simulink model "AttitudeComplementary2"  (Simulink 6.6)
settings: Solver=ode4  StartTime=0.0  StopTime=80  FixedStep=SampleT  RelTol=1e-3
InitFcn:
  | clc
  | Taxi_Var_new
  | failures
  | insInit
  | piccolo_init
values from neighbouring files (symbols this model uses):
  A1 = 0    [Taxi_Var.m]    (also in Taxi_Var_new.m = 0.007)
  Apolar = 0.0899    [Taxi_Var.m]    (also in Taxi_Var_new.m = 0.057)
  APtsamp = 0.005    [failures.m]    (also in piccolo_init.m = 0.05)
  CD0 = 0.0219    [Taxi_Var.m]    (also in Taxi_Var_new.m = 0.022)
  chord = S/span    (= 0.384036716878)    [Taxi_Var.m]    (also in Taxi_Var_new.m = 0.351341681574)
  CL0 = 0.1857    [Taxi_Var.m]    (also in Taxi_Var_new.m = 0.38)
  CLa = 4.6206    [Taxi_Var.m]    (also in Taxi_Var_new.m = 18.5)
  CLa_dot = 1.93    [Taxi_Var.m]    (also in Taxi_Var_new.m = 2.64)
  Clb = -0.0043    [Taxi_Var.m]    (also in Taxi_Var_new.m = -0.06)
  ClDa = 0.1695    [Taxi_Var.m]    (also in Taxi_Var_new.m)
  CLDe = 0.4032    [Taxi_Var.m]    (also in Taxi_Var_new.m = 0.24)
  CLDf = 0.047    [Taxi_Var.m]    (also in Taxi_Var_new.m = 0.4)
  ClDr = 0.0003    [Taxi_Var.m]    (also in Taxi_Var_new.m = 0.055)
  Clp = -0.4425    [Taxi_Var.m]    (also in Taxi_Var_new.m = -0.88)
  CLq = 8.7465    [Taxi_Var.m]    (also in Taxi_Var_new.m = 7.4)
  Clr = 0.0675    [Taxi_Var.m]    (also in Taxi_Var_new.m = 0.04)
  Cm0 = -0.0902    [Taxi_Var.m]    (also in Taxi_Var_new.m = 0.56)
  Cma = -1.3995    [Taxi_Var.m]    (also in Taxi_Var_new.m = -1.58)
  CmDe = -0.9493    [Taxi_Var.m]    (also in Taxi_Var_new.m = -41)
  CmDf = -.021    (= -0.021)    [Taxi_Var.m]    (also in Taxi_Var_new.m)
  Cmq = -10.8760    (= -10.876)    [Taxi_Var.m]    (also in Taxi_Var_new.m = -12)
  Cnb = 0.0281    [Taxi_Var.m]    (also in Taxi_Var_new.m = 0.73)
  CnDa = -0.0031    [Taxi_Var.m]    (also in Taxi_Var_new.m = -0.032)
  CnDr = -0.0882    [Taxi_Var.m]    (also in Taxi_Var_new.m = 0.19)
  Cnp = -0.0695    [Taxi_Var.m]    (also in Taxi_Var_new.m = -0.1)
  Cnr = -0.1045    [Taxi_Var.m]    (also in Taxi_Var_new.m = -0.23)
  CYb = -0.1999    [Taxi_Var.m]    (also in Taxi_Var_new.m = -0.98)
  CYDr = 0.0192    [Taxi_Var.m]    (also in Taxi_Var_new.m = 0.066)
  damax = 25*deg2rad    (= 0.436332312999)    [Taxi_Var.m]    (also in piccolo_init.m)
  damin = -25*deg2rad    (= -0.436332312999)    [Taxi_Var.m]    (also in piccolo_init.m)
  datrim = 0*deg2rad    (= 0)    [Taxi_Var.m]    (also in piccolo_init.m)
  demax = 15*deg2rad    (= 0.261799387799)    [Taxi_Var.m]    (also in piccolo_init.m)
  demin = -15*deg2rad    (= -0.261799387799)    [Taxi_Var.m]    (also in piccolo_init.m)
  detrim = -2.4137*deg2rad    (= -0.0421270121554)    [Taxi_Var.m]    (also in piccolo_init.m = -0.01308996939)
  dfland = 30*deg2rad    (= 0.523598775598)    [Taxi_Var.m]    (also in piccolo_init.m)
  dfmax = 30*deg2rad    (= 0.523598775598)    [Taxi_Var.m]    (also in piccolo_init.m)
  dfmin = 0*deg2rad    (= 0)    [Taxi_Var.m]    (also in piccolo_init.m)
  drmax = 25*deg2rad    (= 0.436332312999)    [Taxi_Var.m]    (also in piccolo_init.m)
  drmin = -25*deg2rad    (= -0.436332312999)    [Taxi_Var.m]    (also in piccolo_init.m)
  drtrim = 0*deg2rad    (= 0)    [Taxi_Var.m]    (also in piccolo_init.m)
  dtmax = 1    [Taxi_Var.m]    (also in piccolo_init.m)
  dtmin = 0    [Taxi_Var.m]    (also in piccolo_init.m)
  dttrim = 0.0725    [Taxi_Var.m]    (also in piccolo_init.m = 0.35)
  Euler_0 = [0; 0; 45]'*pi/180    [Taxi_Var.m]    (also in Taxi_Var_new.m = [0 0 45]'*pi/180)
  heightDown = 0    [insInit.m]
  heightUp = 3000    [insInit.m]
  IdxCmdOrbitRadius = 17    [piccolo_init.m]
  IdxCmdOrbitSense = 18    [piccolo_init.m]
  IdxCmdWp1Alt = 13    [piccolo_init.m]
  IdxCmdWp1Lat = 11    [piccolo_init.m]
  IdxCmdWp1Lon = 12    [piccolo_init.m]
  IdxCmdWp2Alt = 16    [piccolo_init.m]
  IdxCmdWp2Lat = 14    [piccolo_init.m]
  IdxCmdWp2Lon = 15    [piccolo_init.m]
  IdxEstimReserved1 = 4    [piccolo_init.m]
  IdxEstimWEast = 3    [piccolo_init.m]
  IdxEstimWNorth = 2    [piccolo_init.m]
  IdxGainsAltD = 10    [piccolo_init.m]
  IdxGainsAltI = 9    [piccolo_init.m]
  IdxGainsAltP = 8    [piccolo_init.m]
  IdxGainsPdynD = 4    [piccolo_init.m]
  IdxGainsPdynI = 3    [piccolo_init.m]
  IdxGainsPdynP = 2    [piccolo_init.m]
  IdxGainsPitchD = 7    [piccolo_init.m]
  IdxGainsPitchI = 6    [piccolo_init.m]
  IdxGainsPitchP = 5    [piccolo_init.m]
  IdxGainsRollD = 17    [piccolo_init.m]
  IdxGainsRollI = 16    [piccolo_init.m]
  IdxGainsRollP = 15    [piccolo_init.m]
  IdxGainsSlopeElevatorD = 25    [piccolo_init.m]
  IdxGainsSlopeElevatorP = 26    [piccolo_init.m]
  IdxGainsTrackConv = 24    [piccolo_init.m]
  IdxGainsTrackD = 23    [piccolo_init.m]
  IdxGainsTrackI = 22    [piccolo_init.m]
  IdxGainsTrackP = 21    [piccolo_init.m]
  IdxGainsTurnD = 14    [piccolo_init.m]
  IdxGainsTurnI = 13    [piccolo_init.m]
  IdxGainsTurnP = 12    [piccolo_init.m]
  IdxGainsYawD = 20    [piccolo_init.m]
  IdxGainsYawI = 19    [piccolo_init.m]
  IdxGainsYawP = 18    [piccolo_init.m]
  IdxLimitsAileronMax = 11    [piccolo_init.m]
  IdxLimitsAileronMin = 10    [piccolo_init.m]
  IdxLimitsBankMax = 9    [piccolo_init.m]
  IdxLimitsBankMin = 8    [piccolo_init.m]
  IdxLimitsElevatorMax = 13    [piccolo_init.m]
  IdxLimitsElevatorMin = 12    [piccolo_init.m]
  IdxLimitsFlapMax = 19    [piccolo_init.m]
  IdxLimitsFlapMin = 18    [piccolo_init.m]
  IdxLimitsPdynMax = 3    [piccolo_init.m]
  IdxLimitsPdynMin = 2    [piccolo_init.m]
  IdxLimitsRudderMax = 15    [piccolo_init.m]
  IdxLimitsRudderMin = 14    [piccolo_init.m]
  IdxLimitsThrottleMax = 17    [piccolo_init.m]
  IdxLimitsThrottleMin = 16    [piccolo_init.m]
  IdxSensorsAlt = 5    [piccolo_init.m]
  IdxSensorsLat = 3    [piccolo_init.m]
  IdxSensorsLon = 4    [piccolo_init.m]
  IdxSensorsVDown = 8    [piccolo_init.m]
  IdxSensorsVEast = 7    [piccolo_init.m]
  IdxSensorsVNorth = 6    [piccolo_init.m]
  IdxStatesGlobal = 2    [piccolo_init.m]
  IdxStatesManual = 16    [piccolo_init.m]
  IdxStatesMode = 15    [piccolo_init.m]
  ISA_g = 9.815    [Taxi_Var.m]    (also in Taxi_Var_new.m)
  ISA_hmax = 2000    [Taxi_Var.m]    (also in Taxi_Var_new.m)
  ISA_lapse = .0065    (= 0.0065)    [Taxi_Var.m]    (also in Taxi_Var_new.m)
  ISA_P0 = 101325    [Taxi_Var.m]    (also in Taxi_Var_new.m)
  ISA_R = 287    [Taxi_Var.m]    (also in Taxi_Var_new.m)
  ISA_rho0 = 1.225    [Taxi_Var.m]    (also in Taxi_Var_new.m)
  ISA_T0 = 289    [Taxi_Var.m]    (also in Taxi_Var_new.m)
  Ixx = 3.689084    [Taxi_Var.m]    (also in Taxi_Var_new.m = 3.8)
  Iyy = 7.43789    [Taxi_Var.m]    (also in Taxi_Var_new.m = 9.58)
  Izz = 10.22202    [Taxi_Var.m]    (also in Taxi_Var_new.m = 9.68)
  latDown = -100000    [insInit.m]
  latUp = 100000    [insInit.m]
  lonDown = -100000    [insInit.m]
  lonUp = 100000    [insInit.m]
  mass = 22.5    [Taxi_Var.m]    (also in Taxi_Var_new.m = 8.16466266)
  MinThK = 0.075    [Taxi_Var.m]    (also in Taxi_Var_new.m = 0.077)
  ... (+8 more)
undefined symbols (not defined in the file or in its folder): clock, DiscIntNeverNeededParam, Earth, gaind, polesd, WGS84, zerosd
libraries: piccolo_library x60, simulink x51, aerolibconvert2 x14, dspsigops x5, aerolibasang x5, aerolibatmos2 x2, aerolibtransform2 x2, aerolibnav x2, dspmtrx3 x1, aerolibutil x1
(part 4 of 6)

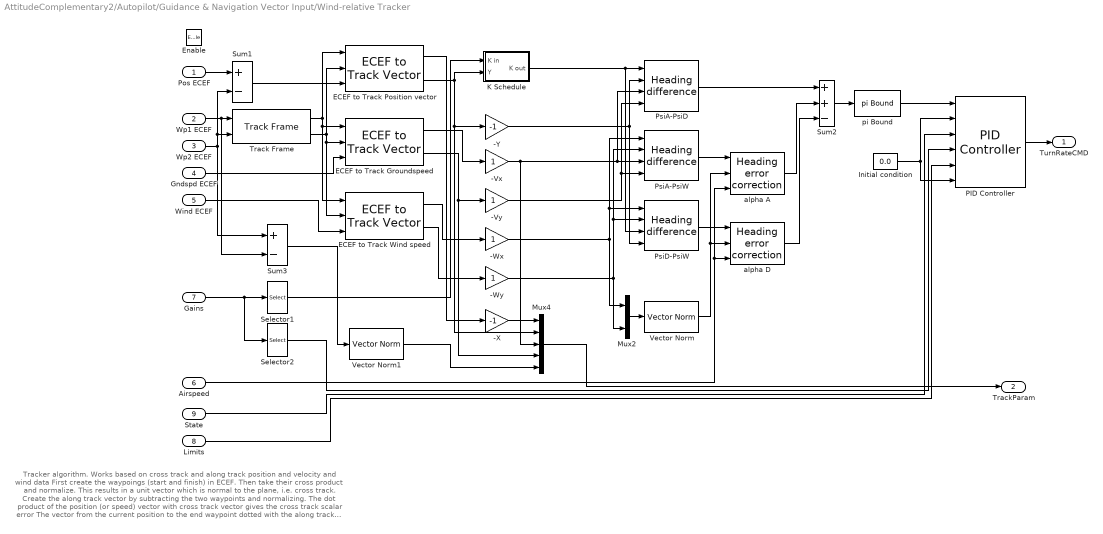
== system AttitudeComplementary2/Autopilot/Guidance & Navigation Vector Input/Wind-relative Tracker ==
  note: Tracker algorithm.  Works based on cross track and along track position and velocity and wind data
      |
      | First create the waypoings (start and finish) in ECEF.  Then take their cross product and normalize.  This results in a unit vector which is normal to the plane, i.e. cross track.
      | Create the along track vector by subtracting the two waypoints and normalizing.
      | The dot product of the position (or speed) vector with cross track vector gives the cross track scalar error
      | The vector from the current position to the end waypoint dotted with the along track vector gives the along track value
  Pos ECEF : Inport
  Wp1 ECEF : Inport  Port=2
  Wp2 ECEF : Inport  Port=3
  Gndspd ECEF : Inport  Port=4
  Wind ECEF : Inport  Port=5
  Airspeed : Inport  Port=6
  Gains : Inport  Port=7
  Limits : Inport  Port=8
  State : Inport  Port=9
  Enable : EnablePort
  -Vx : Gain  SaturateOnIntegerOverflow=on
  -Vy : Gain  SaturateOnIntegerOverflow=on
  -Wx : Gain  SaturateOnIntegerOverflow=on
  -Wy : Gain  SaturateOnIntegerOverflow=on
  -X : Gain  Gain=-1  SaturateOnIntegerOverflow=on
  -Y : Gain  Gain=-1  SaturateOnIntegerOverflow=on
  ECEF to Track Groundspeed : piccolo_library/Transformations/ECEF to Track Vector  SystemSampleTime=-1
  ECEF to Track Position vector : piccolo_library/Transformations/ECEF to Track Vector  SystemSampleTime=-1
  ECEF to Track Wind speed : piccolo_library/Transformations/ECEF to Track Vector  SystemSampleTime=-1
  Initial condition : Constant  Value=0.0
  K Schedule : Subsystem
  Mux2 : Mux  Inputs=2
  Mux4 : Mux  Inputs=5
  PID Controller : piccolo_library/Controllers/PID Controller  SystemSampleTime=-1  tsamp=tsamp  tdelay=tsamp
  PsiA-PsiD : piccolo_library/Controllers/Guidance/Heading difference  SystemSampleTime=-1
  PsiA-PsiW : piccolo_library/Controllers/Guidance/Heading difference  SystemSampleTime=-1
  PsiD-PsiW : piccolo_library/Controllers/Guidance/Heading difference  SystemSampleTime=-1
  Selector1 : Selector  IndexOptions=Index vector (dialog)  Indices=[4]  OutputSizes=1  InputPortWidth=4
  Selector2 : Selector  IndexOptions=Index vector (dialog)  Indices=[1 2 3]  OutputSizes=1  InputPortWidth=4
  Sum1 : Sum  Inputs=+-  SaturateOnIntegerOverflow=on  InputSameDT=on
  Sum2 : Sum  Inputs=++-  SaturateOnIntegerOverflow=on  InputSameDT=on
  Sum3 : Sum  Inputs=+-  SaturateOnIntegerOverflow=on  InputSameDT=on
  Track Frame : piccolo_library/Transformations/Track Frame  SystemSampleTime=-1
  Vector Norm : piccolo_library/Math/Vector Norm  SystemSampleTime=-1
  Vector Norm1 : piccolo_library/Math/Vector Norm  SystemSampleTime=-1
  alpha A : piccolo_library/Controllers/Guidance/Heading error correction  SystemSampleTime=-1
  alpha D : piccolo_library/Controllers/Guidance/Heading error correction  SystemSampleTime=-1
  pi Bound : piccolo_library/Math/pi Bound  SystemSampleTime=-1
  TurnRateCMD : Outport  OutDataType=fixdt(1,16,0)  OutScaling=[]
  TrackParam : Outport  Port=2  OutDataType=fixdt(1,16,0)  OutScaling=[]
  wires:
  Sum3/1 -> Vector Norm1/1
  Vector Norm1/1 -> Mux4/5
  -Y/1 -> PsiD-PsiW/4, PsiA-PsiD/2
  K Schedule/1(K out) -> PsiA-PsiD/1, PsiD-PsiW/3
  PID Controller/1 -> TurnRateCMD/1
  Initial condition/1 -> PID Controller/2, PID Controller/6
  -X/1 -> Mux4/1
  ECEF to Track Wind speed/1 -> -Wx/1
  ECEF to Track Wind speed/2 -> -Wy/1
  ECEF to Track Groundspeed/2 -> Mux4/4, -Vy/1
  ECEF to Track Groundspeed/1 -> -Vx/1
  ECEF to Track Position vector/1 -> -X/1
  ECEF to Track Position vector/2 -> -Y/1, Mux4/2, K Schedule/2(Y)
  Selector1/1 -> K Schedule/1(K in)
  Mux2/1 -> Vector Norm/1
  Vector Norm/1 -> alpha D/2, alpha A/2
  -Wy/1 -> Mux2/2, PsiD-PsiW/2, PsiA-PsiW/2
  -Vy/1 -> PsiA-PsiD/4, PsiA-PsiW/4
  -Wx/1 -> Mux2/1, PsiD-PsiW/1, PsiA-PsiW/1
  -Vx/1 -> Mux4/3, PsiA-PsiD/3, PsiA-PsiW/3
  pi Bound/1 -> PID Controller/1
  Sum2/1 -> pi Bound/1
  alpha D/1 -> Sum2/3
  alpha A/1 -> Sum2/2
  PsiA-PsiD/1 -> Sum2/1
  Limits/1 -> PID Controller/5
  State/1 -> PID Controller/3
  PsiD-PsiW/1 -> alpha D/1
  PsiA-PsiW/1 -> alpha A/1
  Mux4/1 -> TrackParam/1
  Selector2/1 -> PID Controller/4
  Airspeed/1 -> alpha D/3, alpha A/3
  Gains/1 -> Selector2/1, Selector1/1
  Wind ECEF/1 -> ECEF to Track Wind speed/3
  Gndspd ECEF/1 -> ECEF to Track Groundspeed/3
  Track Frame/2 -> ECEF to Track Wind speed/2, ECEF to Track Groundspeed/2, ECEF to Track Position vector/2
  Track Frame/1 -> ECEF to Track Wind speed/1, ECEF to Track Groundspeed/1, ECEF to Track Position vector/1
  Sum1/1 -> ECEF to Track Position vector/3
  Pos ECEF/1 -> Sum1/1
  Wp2 ECEF/1 -> Sum3/1, Sum1/2, Track Frame/2
  Wp1 ECEF/1 -> Sum3/2, Track Frame/1

== system AttitudeComplementary2/Autopilot/Pitch Control  Vector Inputs/PDynCmd ==
  AltError : Inport
  QCmd : Inport  Port=2
  QShift : Inport  Port=3
  QLimits : Inport  Port=4
  States : Inport  Port=5
  Density : Inport  Port=6
  -0.2 : Gain  Gain=-.2  SaturateOnIntegerOverflow=on
  0.3 : Gain  Gain=.3  SaturateOnIntegerOverflow=on
  1-based : Constant  Value=1.1
  All : Constant  Value=0
  Default : Constant  Value=0
  Enabled? : Logic  AllPortsSameDT=off
  Energy or not? : Switch  Threshold=0.5  SaturateOnIntegerOverflow=on
  Gravity : Gain  Gain=9.8  SaturateOnIntegerOverflow=on
  Lateral : Constant
  Limited QShift : piccolo_library/Nonlinear/SaturationEx  SystemSampleTime=-1
  Longitudinal : Constant  Value=0
  Manual assist switch : MultiPortSwitch  Inputs=5  SaturateOnIntegerOverflow=on  InputSameDT=on
  Mux : Mux  Inputs=2
  PDyn saturation : piccolo_library/Nonlinear/SaturationEx  SystemSampleTime=-1
  PDyn saturation1 : piccolo_library/Nonlinear/SaturationEx  SystemSampleTime=-1
  Qshift : Product  SaturateOnIntegerOverflow=on
  Selector1 : Selector  IndexOptions=Index vector (dialog)  Indices=IdxStatesManual  OutputSizes=1  InputPortWidth=SizeStates
  Selector2 : Selector  IndexOptions=Index vector (dialog)  Indices=IdxStatesAltToPdyn  OutputSizes=1  InputPortWidth=SizeStates
  Standard : Constant
  Sum : Sum  Inputs=|++  SaturateOnIntegerOverflow=on
  Sum1 : Sum  SaturateOnIntegerOverflow=on
  QCmdOut : Outport  OutDataType=fixdt(1,16,0)  OutScaling=[]
  QCmdNom : Outport  Port=2  OutDataType=fixdt(1,16,0)  OutScaling=[]
  wires:
  Enabled?/1 -> Energy or not?/2
  Manual assist switch/1 -> Enabled?/1
  Selector2/1 -> Enabled?/2
  PDyn saturation1/1 -> QCmdNom/1
  Sum1/1 -> PDyn saturation/1
  Energy or not?/1 -> Sum1/2
  QLimits/1 -> PDyn saturation1/2, PDyn saturation/2
  PDyn saturation/1 -> QCmdOut/1
  QShift/1 -> Energy or not?/3
  Limited QShift/1 -> Energy or not?/1
  Sum/1 -> Manual assist switch/1
  1-based/1 -> Sum/2
  Selector1/1 -> Sum/1
  States/1 -> Selector2/1, Selector1/1
  Default/1 -> Manual assist switch/6
  All/1 -> Manual assist switch/5
  Lateral/1 -> Manual assist switch/3
  Longitudinal/1 -> Manual assist switch/4
  Standard/1 -> Manual assist switch/2
  QCmd/1 -> PDyn saturation1/1, Sum1/1, -0.2/1, 0.3/1
  Qshift/1 -> Limited QShift/1
  Mux/1 -> Limited QShift/2
  0.3/1 -> Mux/2
  -0.2/1 -> Mux/1
  Gravity/1 -> Qshift/1
  AltError/1 -> Gravity/1
  Density/1 -> Qshift/2

== system AttitudeComplementary2/Autopilot/Pitch Control  Vector Inputs/Pdyn Hold ==
  Input : Inport
  Cmd : Inport  Port=2
  State : Inport  Port=3
  Gains : Inport  Port=4
  Limits : Inport  Port=5
  Actuator Trim : Inport  Port=6
  50 [Pa/s] : Constant  Value=100
  PID Controller : Subsystem  AncestorBlock=piccolo_library/Controllers/PID Controller  mask(PID Controller){tsamp=tsamp, tdelay=0.5}
      mask prompts: tsamp "Sample time:"; tdelay "Time derivative delay:"
      mask help: Generic PID (proportional, integral, derivative) controller with a single input and a single output.
  Rate Limit Ex : piccolo_library/Nonlinear/Rate Limit Ex  SystemSampleTime=-1  T=tsamp
  Out : Outport  OutDataType=fixdt(1,16,0)  OutScaling=[]
  wires:
  Actuator Trim/1 -> PID Controller/6(IniCond)
  Limits/1 -> PID Controller/5(Limits)
  Gains/1 -> PID Controller/4(Gains)
  State/1 -> PID Controller/3(State)
  PID Controller/1(Output) -> Out/1
  Rate Limit Ex/1 -> PID Controller/2(Cmd)
  Input/1 -> PID Controller/1(Input)
  50 [Pa/s]/1 -> Rate Limit Ex/2
  Cmd/1 -> Rate Limit Ex/1

== system AttitudeComplementary2/Autopilot/Pitch Control  Vector Inputs/Pitch Angle Hold ==
  note: Controller which takes in pitch rate and pitch angle and outputs elevator. The integral term is not used. Yet.
  Pitch angle : Inport
  Pitch rate : Inport  Port=2
  Pitch angle cmd : Inport  Port=3
  Pitch rate cmd : Inport  Port=4
  State : Inport  Port=5
  Gains : Inport  Port=6
  Demux1 : Demux  Outputs=3
  Demux5 : Demux  Outputs=3
  Derivative Gain : Product  Inputs=3  SaturateOnIntegerOverflow=on  InputSameDT=on
  Low-pass Filter : piccolo_library/Filters/Low-pass Filter  SystemSampleTime=-1  f=3  t=tsamp
  Proportional Gain : Product  Inputs=3  SaturateOnIntegerOverflow=on  InputSameDT=on
  Scope : Scope  NumInputPorts=5
      settings: YMin=-1~-0.075~-0.075~-5e+006~-5e+006  YMax=1~0.1~0.1~3.5e+007~3.5e+007  SaveName=ScopeData5
  Sum : Sum  SaturateOnIntegerOverflow=on  InputSameDT=on
  Sum1 : Sum  Inputs=|+-  SaturateOnIntegerOverflow=on  InputSameDT=on
  Sum2 : Sum  Inputs=|+-  SaturateOnIntegerOverflow=on  InputSameDT=on
  Terminator : Terminator
  Terminator1 : Terminator
  Out : Outport  OutDataType=fixdt(1,16,0)  OutScaling=[]
  wires:
  Demux1/2 -> Terminator1/1
  Demux1/1 -> Proportional Gain/3
  Demux1/3 -> Derivative Gain/3
  State/1 -> Demux1/1
  Demux5/2 -> Terminator/1
  Sum/1 -> Out/1, Scope/4
  Derivative Gain/1 -> Sum/2
  Proportional Gain/1 -> Sum/1, Scope/5
  Demux5/3 -> Derivative Gain/2
  Low-pass Filter/1 -> Derivative Gain/1
  Demux5/1 -> Proportional Gain/2
  Sum2/1 -> Proportional Gain/1, Scope/3
  Sum1/1 -> Low-pass Filter/1
  Pitch angle cmd/1 -> Sum2/2, Scope/1
  Pitch angle/1 -> Sum2/1, Scope/2
  Gains/1 -> Demux5/1
  Pitch rate/1 -> Sum1/1
  Pitch rate cmd/1 -> Sum1/2

== system AttitudeComplementary2/Autopilot/Roll Control Vector Inputs/Bank Angle Hold ==
  note: Controller which takes in roll rate and roll angle and outputs aileron.  Note that the derivative
      | term is simply the roll rate rather than the derivative of the error signal.
      | This is for backward compatible systems which aren't using the attitude data.
  note: pid
  Roll Rate : Inport
  Roll Angle : Inport  Port=2
  Cmd : Inport  Port=3
  State : Inport  Port=4
  Gains : Inport  Port=5
  Limits : Inport  Port=6
  IniCond : Inport  Port=7
  Demux1 : Demux  Outputs=3
  Demux2 : Demux  Outputs=3
  Derivative Gain : Product  Inputs=3  SaturateOnIntegerOverflow=on  InputSameDT=on
  Extended Integrator : piccolo_library/Integrators/Extended Integrator  SystemSampleTime=-1  T=tsamp
  Low-pass Filter : piccolo_library/Filters/Low-pass Filter  SystemSampleTime=-1  f=3  t=tsamp
  Proportional Gain : Product  Inputs=3  SaturateOnIntegerOverflow=on  InputSameDT=on
  Scope : Scope  NumInputPorts=10
      settings: YMin=-1~-0.07~-0.07~-0.02~-1~-1~-1~-1~-1~-1  YMax=1~0.03~0.03~0.07~1~1~1~1~1~1
  Sum2 : Sum  Inputs=+++  SaturateOnIntegerOverflow=on  InputSameDT=on
  Sum3 : Sum  Inputs=|+-  SaturateOnIntegerOverflow=on  InputSameDT=on
  Out : Outport  OutDataType=fixdt(1,16,0)  OutScaling=[]
  wires:
  Demux2/3 -> Derivative Gain/3
  Demux2/2 -> Extended Integrator/3
  Demux2/1 -> Proportional Gain/3
  State/1 -> Demux2/1
  Roll Rate/1 -> Low-pass Filter/1
  Low-pass Filter/1 -> Derivative Gain/1
  Demux1/2 -> Extended Integrator/4
  Sum2/1 -> Out/1, Scope/4
  Derivative Gain/1 -> Sum2/3, Scope/6  "derv"
  Extended Integrator/1 -> Sum2/2, Scope/5  "int"
  Proportional Gain/1 -> Sum2/1
  Demux1/3 -> Derivative Gain/2
  Demux1/1 -> Proportional Gain/2
  Limits/1 -> Extended Integrator/5
  IniCond/1 -> Extended Integrator/2
  Sum3/1 -> Extended Integrator/1, Proportional Gain/1, Scope/3  "err"
  Gains/1 -> Demux1/1
  Roll Angle/1 -> Scope/2, Sum3/1  "roll"
  Cmd/1 -> Sum3/2, Scope/1  "cmd"

== system AttitudeComplementary2/Autopilot/Roll Control Vector Inputs/Damper switch ==
  note: Select whether the individual components of the pitch and roll damper  loops are enabled or disabled.
      | This is done based on the specific loop enable state, the global state, and the mode of the autopilot.
      |
      | Note the use of the multiport  switch.  This switch is one based, and will truncate floating point
      | numbers.  Hence we add by 1.1 to guarantee we don't get the wrong state based on rounding
      | error.
  Globals : Inport
  Loop : Inport  Port=2
  Climbout : Constant
  Convert to 1 based : Constant  Value=1.1
  Default : Constant
  Demux : Demux  Outputs=3
  Display1 : Display
  Display2 : Display
  Display3 : Display
  Final Approach : Constant
  Flying : Constant
  Global and Loop on/off : Product  SaturateOnIntegerOverflow=on
  Land pattern : Constant
  Loop on or off : Switch  Threshold=0.5  SaturateOnIntegerOverflow=on
  Mux : Mux  Inputs=3
  Mux1 : Mux  Inputs=3
  Pre launch : Constant  Value=0
  Proportional\ Integral switch : MultiPortSwitch  Inputs=8  SaturateOnIntegerOverflow=on  InputSameDT=on
  Sum : Sum  Inputs=++|  SaturateOnIntegerOverflow=on  InputSameDT=on
  Terminator : Terminator
  Touchdown : Constant
  Transition : Constant  Value=0
  Zero : Constant  Value=0
  TriOut : Outport  OutDataType=fixdt(1,16,0)  OutScaling=[]
  wires:
  Default/1 -> Proportional\ Integral switch/9
  Touchdown/1 -> Proportional\ Integral switch/8
  Demux/3 -> Terminator/1
  Mux1/1 -> Loop on or off/1
  Proportional\ Integral switch/1 -> Mux1/3, Mux1/2, Mux1/1
  Final Approach/1 -> Proportional\ Integral switch/7
  Land pattern/1 -> Proportional\ Integral switch/6
  Flying/1 -> Proportional\ Integral switch/5
  Transition/1 -> Proportional\ Integral switch/3
  Climbout/1 -> Proportional\ Integral switch/4
  Pre launch/1 -> Proportional\ Integral switch/2
  Convert to 1 based/1 -> Sum/1
  Demux/2 -> Sum/2
  Sum/1 -> Proportional\ Integral switch/1
  Global and Loop on/off/1 -> Loop on or off/2, Display2/1
  Loop/1 -> Global and Loop on/off/2, Display3/1
  Demux/1 -> Global and Loop on/off/1, Display1/1
  Globals/1 -> Demux/1
  Zero/1 -> Mux/3, Mux/2, Mux/1
  Mux/1 -> Loop on or off/3
  Loop on or off/1 -> TriOut/1

== system AttitudeComplementary2/Autopilot/Roll Control Vector Inputs/Turn Rate Hold ==
  note: Standard PID feedback controller with integrator saturation. There are three gains, and three states, one for each term
  Input : Inport
  Cmd : Inport  Port=2
  State : Inport  Port=3
  Gains : Inport  Port=4
  Limits : Inport  Port=5
  IniCond : Inport  Port=6
  Demux : Demux  Outputs=3
  Demux1 : Demux  Outputs=3
  Derivative Gain : Product  Inputs=3  SaturateOnIntegerOverflow=on  InputSameDT=on
  Extended Integrator : piccolo_library/Integrators/Extended Integrator  SystemSampleTime=-1  T=tsamp
  Proportional Gain : Product  Inputs=3  SaturateOnIntegerOverflow=on  InputSameDT=on
  Scope1 : Scope  NumInputPorts=5
      settings: YMin=0.09325~0.09~-0.005~-1~-1  YMax=0.09475~0.1075~0.0125~1~1  SaveName=ScopeData25
  Sum : Sum  Inputs=|+-  SaturateOnIntegerOverflow=on
  Sum3 : Sum  Inputs=+++  SaturateOnIntegerOverflow=on  InputSameDT=on
  dx/dt with TD : piccolo_library/Derivatives/dx//dt with TD  SystemSampleTime=-1  tsamp=tsamp  tdelay=tdelay
  Output : Outport  OutDataType=fixdt(1,16,0)  OutScaling=[]
  wires:
  Sum3/1 -> Output/1, Scope1/4
  Demux1/3 -> Derivative Gain/3
  Demux1/2 -> Extended Integrator/3
  Demux1/1 -> Proportional Gain/3
  State/1 -> Demux1/1
  IniCond/1 -> Extended Integrator/2
  Limits/1 -> Extended Integrator/5
  Demux/2 -> Extended Integrator/4
  Extended Integrator/1 -> Sum3/2
  Derivative Gain/1 -> Sum3/3
  Proportional Gain/1 -> Sum3/1
  Demux/3 -> Derivative Gain/2
  Demux/1 -> Proportional Gain/2
  Gains/1 -> Demux/1
  dx/dt with TD/1 -> Derivative Gain/1
  Sum/1 -> Extended Integrator/1, dx/dt with TD/1, Scope1/3, Proportional Gain/1
  Cmd/1 -> Sum/2, Scope1/1
  Input/1 -> Sum/1, Scope1/2

== system AttitudeComplementary2/Get GPS in LTP/Geod2LTP2/ECEF2LTP (UEN) ==
  ECEF coordinates : Inport
  "Long, Lat" : Inport  Port=2
  Deg2R : Gain  Gain=pi/180  SaturateOnIntegerOverflow=on
  Demux3 : Demux  Outputs=2
  From Body to Universal1 : Subsystem
  Product1 : Product  Multiplication=Matrix(*)  SaturateOnIntegerOverflow=on  InputSameDT=on
  Out : Outport
  wires:
  "Long, Lat"/1 -> Deg2R/1
  Product1/1 -> Out/1
  Demux3/2 -> From Body to Universal1/2(lat)
  Demux3/1 -> From Body to Universal1/1(long)
  Deg2R/1 -> Demux3/1
  ECEF coordinates/1 -> Product1/2
  From Body to Universal1/1(DCM) -> Product1/1

== system AttitudeComplementary2/Get GPS in LTP/Geod2LTP2/Geod2ECEF ==
  "height, m" : Inport
  "lat, deg" : Inport  Port=2
  lon,deg : Inport  Port=3
  (Rh+h)cos(phi)*cos(lamb)=Xe : Product  Inputs=3  SaturateOnIntegerOverflow=on  InputSameDT=on
  (Rh+h)cos(phi)*sin(lamb)=Ye : Product  Inputs=3  SaturateOnIntegerOverflow=on  InputSameDT=on
  Deg2R : Gain  Gain=pi/180  SaturateOnIntegerOverflow=on
  "Deg2R " : Gain  Gain=pi/180  SaturateOnIntegerOverflow=on
  Product1 : Product  SaturateOnIntegerOverflow=on  InputSameDT=on
  Re=equatorial radius : Constant  Value=Re
  Rh : Product  Inputs=*/  SaturateOnIntegerOverflow=on  InputSameDT=on
  Rh(1-e^2) : Product  SaturateOnIntegerOverflow=on  InputSameDT=on
  Sum1 : Sum  Inputs=+-|  SaturateOnIntegerOverflow=on  InputSameDT=on
  Sum2 : Sum  SaturateOnIntegerOverflow=on  InputSameDT=on
      settings: AttributesFormatString=Rh+h
  Sum3 : Sum  Inputs=|+-  SaturateOnIntegerOverflow=on  InputSameDT=on
  Sum4 : Sum  SaturateOnIntegerOverflow=on  InputSameDT=on
      settings: AttributesFormatString=(1-e^2)Rh+h
  Ze : Product  SaturateOnIntegerOverflow=on  InputSameDT=on
  const : Constant
  const1 : Constant
  cos(lamb) : Trigonometry  Operator=cos
  cos(phi) : Trigonometry  Operator=cos
  eccentricity^2 : Subsystem
  f : Fcn  Expr=sqrt(u(1))
  sin(lamb) : Trigonometry
  sin(phi) : Trigonometry
  sin(phi)^2 : Product  SaturateOnIntegerOverflow=on  InputSameDT=on
  "Xe, m " : Outport
  "Ye, m " : Outport  Port=2
  "Ze, m " : Outport  Port=3
  wires:
  "lat, deg"/1 -> Deg2R/1
  sin(phi)/1 -> sin(phi)^2/1, sin(phi)^2/2, Ze/1
  f/1 -> Rh/2
  Re=equatorial radius/1 -> Rh/1
  Rh/1 -> Sum2/2, Rh(1-e^2)/2
  Product1/1 -> Sum1/2
  Sum1/1 -> f/1
  const/1 -> Sum1/1
  "height, m"/1 -> Sum4/2, Sum2/1
  eccentricity^2/1(e^2) -> Product1/1, Sum3/2
  sin(phi)^2/1 -> Product1/2
  const1/1 -> Sum3/1
  Sum3/1 -> Rh(1-e^2)/1  "1-e^2"
  Rh(1-e^2)/1 -> Sum4/1
  Sum4/1 -> Ze/2
  lon,deg/1 -> "Deg2R "/1
  cos(phi)/1 -> (Rh+h)cos(phi)*cos(lamb)=Xe/2, (Rh+h)cos(phi)*sin(lamb)=Ye/2
  cos(lamb)/1 -> (Rh+h)cos(phi)*cos(lamb)=Xe/3
  sin(lamb)/1 -> (Rh+h)cos(phi)*sin(lamb)=Ye/3
  Ze/1 -> "Ze, m "/1
  Deg2R/1 -> cos(phi)/1, sin(phi)/1
  "Deg2R "/1 -> cos(lamb)/1, sin(lamb)/1
  Sum2/1 -> (Rh+h)cos(phi)*sin(lamb)=Ye/1, (Rh+h)cos(phi)*cos(lamb)=Xe/1
  (Rh+h)cos(phi)*cos(lamb)=Xe/1 -> "Xe, m "/1
  (Rh+h)cos(phi)*sin(lamb)=Ye/1 -> "Ye, m "/1

== system AttitudeComplementary2/Get GPS in LTP/Geod2LTP2/Geod2ECEF1 ==
  "height, m" : Inport
  "lat, deg" : Inport  Port=2
  lon,deg : Inport  Port=3
  (Rh+h)cos(phi)*cos(lamb)=Xe : Product  Inputs=3  SaturateOnIntegerOverflow=on  InputSameDT=on
  (Rh+h)cos(phi)*sin(lamb)=Ye : Product  Inputs=3  SaturateOnIntegerOverflow=on  InputSameDT=on
  Deg2R : Gain  Gain=pi/180  SaturateOnIntegerOverflow=on
  "Deg2R " : Gain  Gain=pi/180  SaturateOnIntegerOverflow=on
  Product1 : Product  SaturateOnIntegerOverflow=on  InputSameDT=on
  Re=equatorial radius : Constant  Value=Re
  Rh : Product  Inputs=*/  SaturateOnIntegerOverflow=on  InputSameDT=on
  Rh(1-e^2) : Product  SaturateOnIntegerOverflow=on  InputSameDT=on
  Sum1 : Sum  Inputs=+-|  SaturateOnIntegerOverflow=on  InputSameDT=on
  Sum2 : Sum  SaturateOnIntegerOverflow=on  InputSameDT=on
      settings: AttributesFormatString=Rh+h
  Sum3 : Sum  Inputs=|+-  SaturateOnIntegerOverflow=on  InputSameDT=on
  Sum4 : Sum  SaturateOnIntegerOverflow=on  InputSameDT=on
      settings: AttributesFormatString=(1-e^2)Rh+h
  Ze : Product  SaturateOnIntegerOverflow=on  InputSameDT=on
  const : Constant
  const1 : Constant
  cos(lamb) : Trigonometry  Operator=cos
  cos(phi) : Trigonometry  Operator=cos
  eccentricity^2 : Subsystem
  f : Fcn  Expr=sqrt(u(1))
  sin(lamb) : Trigonometry
  sin(phi) : Trigonometry
  sin(phi)^2 : Product  SaturateOnIntegerOverflow=on  InputSameDT=on
  "Xe, m " : Outport
  "Ye, m " : Outport  Port=2
  "Ze, m " : Outport  Port=3
  wires:
  (Rh+h)cos(phi)*sin(lamb)=Ye/1 -> "Ye, m "/1
  (Rh+h)cos(phi)*cos(lamb)=Xe/1 -> "Xe, m "/1
  Sum2/1 -> (Rh+h)cos(phi)*cos(lamb)=Xe/1, (Rh+h)cos(phi)*sin(lamb)=Ye/1
  "Deg2R "/1 -> sin(lamb)/1, cos(lamb)/1
  Deg2R/1 -> sin(phi)/1, cos(phi)/1
  Ze/1 -> "Ze, m "/1
  sin(lamb)/1 -> (Rh+h)cos(phi)*sin(lamb)=Ye/3
  cos(lamb)/1 -> (Rh+h)cos(phi)*cos(lamb)=Xe/3
  cos(phi)/1 -> (Rh+h)cos(phi)*sin(lamb)=Ye/2, (Rh+h)cos(phi)*cos(lamb)=Xe/2
  lon,deg/1 -> "Deg2R "/1
  Sum4/1 -> Ze/2
  Rh(1-e^2)/1 -> Sum4/1
  Sum3/1 -> Rh(1-e^2)/1  "1-e^2"
  const1/1 -> Sum3/1
  sin(phi)^2/1 -> Product1/2
  eccentricity^2/1(e^2) -> Sum3/2, Product1/1
  "height, m"/1 -> Sum2/1, Sum4/2
  const/1 -> Sum1/1
  Sum1/1 -> f/1
  Product1/1 -> Sum1/2
  Rh/1 -> Rh(1-e^2)/2, Sum2/2
  Re=equatorial radius/1 -> Rh/1
  f/1 -> Rh/2
  sin(phi)/1 -> Ze/1, sin(phi)^2/2, sin(phi)^2/1
  "lat, deg"/1 -> Deg2R/1

== system AttitudeComplementary2/Gyro Comp/3vector LPF/Low Pass1 ==
  In1 : Inport
  Discrete Zero-Pole : DiscreteZeroPole  Zeros=zerosd  Poles=polesd  Gain=gaind  SampleTime=SampleTime
  Out1 : Outport
  wires:
  In1/1 -> Discrete Zero-Pole/1
  Discrete Zero-Pole/1 -> Out1/1

== system AttitudeComplementary2/Gyro Comp/3vector LPF/Low Pass2 ==
  In1 : Inport
  Discrete Zero-Pole : DiscreteZeroPole  Zeros=zerosd  Poles=polesd  Gain=gaind  SampleTime=SampleTime
  Out1 : Outport
  wires:
  Discrete Zero-Pole/1 -> Out1/1
  In1/1 -> Discrete Zero-Pole/1

== system AttitudeComplementary2/Gyro Comp/3vector LPF/Low Pass3 ==
  In1 : Inport
  Discrete Zero-Pole : DiscreteZeroPole  Zeros=zerosd  Poles=polesd  Gain=gaind  SampleTime=SampleTime
  Out1 : Outport
  wires:
  In1/1 -> Discrete Zero-Pole/1
  Discrete Zero-Pole/1 -> Out1/1

== system AttitudeComplementary2/Interpolate Data/Subsystem/Clock Updates ==
  change? : Inport
  Constant : Constant
  Constant1 : Constant  Value=0
  Constant2 : Constant  Value=SampleT
  Discrete-Time Integrator : DiscreteIntegrator  ExternalReset=rising  InitialConditionSource=external  SampleTime=SampleT  ICPrevOutput=DiscIntNeverNeededParam  ICPrevScaledInput=DiscIntNeverNeededParam
  Integer Delay2 : simulink/Discrete/Integer Delay  vinit=0.0  samptime=-1  NumDelays=1
  Sum : Sum  Inputs=|++
  clock : Outport
  wires:
  Constant/1 -> Discrete-Time Integrator/1
  Constant1/1 -> Discrete-Time Integrator/3
  Discrete-Time Integrator/1 -> Integer Delay2/1
  change?/1 -> Discrete-Time Integrator/2
  Integer Delay2/1 -> Sum/1
  Constant2/1 -> Sum/2
  Sum/1 -> clock/1

== system AttitudeComplementary2/Interpolate Data/Subsystem/Detect Change ==
  Data : Inport
  Abs1 : Abs
  Difference1 : simulink/Discrete/Difference  SystemSampleTime=-1  ICPrevInput=0.0  OutDataType=sfix(16)  OutScaling=2^-10  DoSatur=off
  Saturation1 : Saturate  UpperLimit=1  LowerLimit=0  SampleTime=SampleT
  change? : Outport
  wires:
  Difference1/1 -> Abs1/1
  Abs1/1 -> Saturation1/1
  Data/1 -> Difference1/1
  Saturation1/1 -> change?/1

== system AttitudeComplementary2/Interpolate Data/Subsystem/Generate Clock ==
  Reset : Inport
  Constant : Constant
  Discrete-Time Integrator : DiscreteIntegrator  ExternalReset=rising  InitialConditionMode=State only (most efficient)  SampleTime=SampleT  ICPrevOutput=DiscIntNeverNeededParam  ICPrevScaledInput=DiscIntNeverNeededParam
  Rate Transition2 : RateTransition  OutPortSampleTime=SampleT
  Clock : Outport
  wires:
  Constant/1 -> Discrete-Time Integrator/1
  Rate Transition2/1 -> Discrete-Time Integrator/2
  Reset/1 -> Rate Transition2/1
  Discrete-Time Integrator/1 -> Clock/1

== system AttitudeComplementary2/Interpolate Data/Subsystem/Low Pass ==
  In1 : Inport
  Discrete Zero-Pole : DiscreteZeroPole  Zeros=zerosd  Poles=polesd  Gain=gaind  SampleTime=SampleTime
  Out1 : Outport
  wires:
  Discrete Zero-Pole/1 -> Out1/1
  In1/1 -> Discrete Zero-Pole/1

== system AttitudeComplementary2/Interpolate Data/Subsystem/Low Pass1 ==
  In1 : Inport
  Discrete Zero-Pole : DiscreteZeroPole  Zeros=zerosd  Poles=polesd  Gain=gaind  SampleTime=SampleTime
  Out1 : Outport
  wires:
  In1/1 -> Discrete Zero-Pole/1
  Discrete Zero-Pole/1 -> Out1/1

== system AttitudeComplementary2/Interpolate Data/Subsystem/Low Pass2 ==
  In1 : Inport
  Discrete Zero-Pole : DiscreteZeroPole  Zeros=zerosd  Poles=polesd  Gain=gaind  SampleTime=SampleTime
  Out1 : Outport
  wires:
  Discrete Zero-Pole/1 -> Out1/1
  In1/1 -> Discrete Zero-Pole/1

== system AttitudeComplementary2/Interpolate Data/Subsystem/SampleData ==
  data : Inport
  clock : Inport  Port=2
  Enable : EnablePort
  Integer Delay{,1..3} (4 alike) : simulink/Discrete/Integer Delay  vinit=0.0  samptime=-1  NumDelays=1
  k : Outport
  km1 : Outport  Port=2
  km2 : Outport  Port=3
  tm1 : Outport  Port=4
  tm2 : Outport  Port=5
  wires:
  data/1 -> Integer Delay/1, k/1
  Integer Delay/1 -> Integer Delay1/1, km1/1
  Integer Delay1/1 -> km2/1
  clock/1 -> Integer Delay2/1
  Integer Delay2/1 -> tm1/1, Integer Delay3/1
  Integer Delay3/1 -> tm2/1

== system AttitudeComplementary2/Interpolate Data/Subsystem1/Detect Change ==
  Data : Inport
  Abs1 : Abs
  Difference1 : simulink/Discrete/Difference  SystemSampleTime=-1  ICPrevInput=0.0  OutDataType=sfix(16)  OutScaling=2^-10  DoSatur=off
  Saturation1 : Saturate  UpperLimit=1  LowerLimit=0  SampleTime=SampleT
  change? : Outport
  wires:
  Saturation1/1 -> change?/1
  Data/1 -> Difference1/1
  Abs1/1 -> Saturation1/1
  Difference1/1 -> Abs1/1

== system AttitudeComplementary2/Interpolate Data/Subsystem1/Generate Clock ==
  Reset : Inport
  Constant : Constant
  Discrete-Time Integrator : DiscreteIntegrator  ExternalReset=rising  InitialConditionMode=State only (most efficient)  SampleTime=SampleT  ICPrevOutput=DiscIntNeverNeededParam  ICPrevScaledInput=DiscIntNeverNeededParam
  Rate Transition2 : RateTransition  OutPortSampleTime=SampleT
  Clock : Outport
  wires:
  Discrete-Time Integrator/1 -> Clock/1
  Reset/1 -> Rate Transition2/1
  Rate Transition2/1 -> Discrete-Time Integrator/2
  Constant/1 -> Discrete-Time Integrator/1

== system AttitudeComplementary2/Interpolate Data/Subsystem1/Low Pass ==
  In1 : Inport
  Discrete Zero-Pole : DiscreteZeroPole  Zeros=zerosd  Poles=polesd  Gain=gaind  SampleTime=SampleTime
  Out1 : Outport
  wires:
  In1/1 -> Discrete Zero-Pole/1
  Discrete Zero-Pole/1 -> Out1/1

== system AttitudeComplementary2/Interpolate Data/Subsystem1/Low Pass1 ==
  In1 : Inport
  Discrete Zero-Pole : DiscreteZeroPole  Zeros=zerosd  Poles=polesd  Gain=gaind  SampleTime=SampleTime
  Out1 : Outport
  wires:
  Discrete Zero-Pole/1 -> Out1/1
  In1/1 -> Discrete Zero-Pole/1

== system AttitudeComplementary2/Interpolate Data/Subsystem1/SampleData ==
  data : Inport
  Enable : EnablePort
  Integer Delay : simulink/Discrete/Integer Delay  vinit=0.0  samptime=-1  NumDelays=1
  Integer Delay1 : simulink/Discrete/Integer Delay  vinit=0.0  samptime=-1  NumDelays=1
  k : Outport
  km1 : Outport  Port=2
  km2 : Outport  Port=3
  wires:
  Integer Delay1/1 -> km2/1
  Integer Delay/1 -> km1/1, Integer Delay1/1
  data/1 -> k/1, Integer Delay/1

== system AttitudeComplementary2/Interpolate Data/Subsystem2/Detect Change ==
  Data : Inport
  Abs1 : Abs
  Difference1 : simulink/Discrete/Difference  SystemSampleTime=-1  ICPrevInput=0.0  OutDataType=sfix(16)  OutScaling=2^-10  DoSatur=off
  Saturation1 : Saturate  UpperLimit=1  LowerLimit=0  SampleTime=SampleT
  change? : Outport
  wires:
  Difference1/1 -> Abs1/1
  Abs1/1 -> Saturation1/1
  Data/1 -> Difference1/1
  Saturation1/1 -> change?/1

== system AttitudeComplementary2/Interpolate Data/Subsystem2/Generate Clock ==
  Reset : Inport
  Constant : Constant
  Discrete-Time Integrator : DiscreteIntegrator  ExternalReset=rising  InitialConditionMode=State only (most efficient)  SampleTime=SampleT  ICPrevOutput=DiscIntNeverNeededParam  ICPrevScaledInput=DiscIntNeverNeededParam
  Rate Transition2 : RateTransition  OutPortSampleTime=SampleT
  Clock : Outport
  wires:
  Constant/1 -> Discrete-Time Integrator/1
  Rate Transition2/1 -> Discrete-Time Integrator/2
  Reset/1 -> Rate Transition2/1
  Discrete-Time Integrator/1 -> Clock/1

== system AttitudeComplementary2/Interpolate Data/Subsystem2/Low Pass ==
  In1 : Inport
  Discrete Zero-Pole : DiscreteZeroPole  Zeros=zerosd  Poles=polesd  Gain=gaind  SampleTime=SampleTime
  Out1 : Outport
  wires:
  Discrete Zero-Pole/1 -> Out1/1
  In1/1 -> Discrete Zero-Pole/1

== system AttitudeComplementary2/Interpolate Data/Subsystem2/Low Pass1 ==
  In1 : Inport
  Discrete Zero-Pole : DiscreteZeroPole  Zeros=zerosd  Poles=polesd  Gain=gaind  SampleTime=SampleTime
  Out1 : Outport
  wires:
  In1/1 -> Discrete Zero-Pole/1
  Discrete Zero-Pole/1 -> Out1/1

== system AttitudeComplementary2/Interpolate Data/Subsystem2/SampleData ==
  data : Inport
  Enable : EnablePort
  Integer Delay : simulink/Discrete/Integer Delay  vinit=0.0  samptime=-1  NumDelays=1
  Integer Delay1 : simulink/Discrete/Integer Delay  vinit=0.0  samptime=-1  NumDelays=1
  k : Outport
  km1 : Outport  Port=2
  km2 : Outport  Port=3
  wires:
  data/1 -> Integer Delay/1, k/1
  Integer Delay/1 -> Integer Delay1/1, km1/1
  Integer Delay1/1 -> km2/1

== system AttitudeComplementary2/L1 Adaptive Controller LATERAL-DIRECTIONAL/PF Yaw Channel L1 Augmentation/Adaptive Law ==
  u_psi_tilda : Inport
  Integrator : Integrator  LimitOutput=on  UpperSaturationLimit=Pbound  LowerSaturationLimit=-Pbound
  ON : Constant  Value=gamma
  Projection : Product  RndMeth=Zero
  Scope1 : Scope  NumInputPorts=3
      settings: YMin=-0.1~-0.004~-6  YMax=0.1~0.003~8  SaveName=ScopeData27
  sighat_2 : Outport
  wires:
  Integrator/1 -> sighat_2/1, Scope1/1
  ON/1 -> Projection/1
  Projection/1 -> Integrator/1, Scope1/3
  u_psi_tilda/1 -> Projection/2, Scope1/2  "u_psi_tilda"

== system AttitudeComplementary2/L1 Adaptive Controller LATERAL-DIRECTIONAL/PF Yaw Channel L1 Augmentation/C(s) ==
  sighat_2 : Inport
  Integrator2 : Integrator
  ON : Constant  Value=omega
  Product : Product  RndMeth=Zero
  Sum2 : Sum  Inputs=|+-
  C_sighat_2 : Outport
  wires:
  Integrator2/1 -> C_sighat_2/1, Sum2/2
  Sum2/1 -> Product/2
  Product/1 -> Integrator2/1
  sighat_2/1 -> Sum2/1
  ON/1 -> Product/1

== system AttitudeComplementary2/L1 Adaptive Controller LATERAL-DIRECTIONAL/PF Yaw Channel L1 Augmentation/State predictor ==
  u2 : Inport
  sighat_2 : Inport  Port=2
  Integrator2 : Integrator
  ON : Constant  Value=m
  Product : Product  RndMeth=Zero
  Sum1 : Sum  Inputs=|++
  Sum2 : Sum  Inputs=|+-
  u_psi_hat : Outport
  wires:
  sighat_2/1 -> Sum1/2
  Sum1/1 -> Sum2/1
  u2/1 -> Sum1/1
  Integrator2/1 -> u_psi_hat/1, Sum2/2
  Sum2/1 -> Product/2
  Product/1 -> Integrator2/1
  ON/1 -> Product/1

== system AttitudeComplementary2/L1 Adaptive Controller LONGITUDINAL/PF Yaw Channel L1 Augmentation/Adaptive Law ==
  u_psi_tilda : Inport
  Integrator : Integrator  LimitOutput=on  UpperSaturationLimit=Pbound  LowerSaturationLimit=-Pbound
  ON : Constant  Value=gamma
  Projection : Product  RndMeth=Zero
  Scope1 : Scope  NumInputPorts=3
      settings: TimeRange=4  YMin=-0.1~-1000~-6  YMax=0.1~200~8  SaveName=ScopeData27
  sighat_2 : Outport
  wires:
  u_psi_tilda/1 -> Scope1/2, Projection/2  "u_psi_tilda"
  Projection/1 -> Scope1/3, Integrator/1
  ON/1 -> Projection/1
  Integrator/1 -> Scope1/1, sighat_2/1

== system AttitudeComplementary2/L1 Adaptive Controller LONGITUDINAL/PF Yaw Channel L1 Augmentation/C(s) ==
  sighat_2 : Inport
  Integrator2 : Integrator
  ON : Constant  Value=omega
  Product : Product  RndMeth=Zero
  Sum2 : Sum  Inputs=|+-
  C_sighat_2 : Outport
  wires:
  ON/1 -> Product/1
  sighat_2/1 -> Sum2/1
  Product/1 -> Integrator2/1
  Sum2/1 -> Product/2
  Integrator2/1 -> Sum2/2, C_sighat_2/1

== system AttitudeComplementary2/L1 Adaptive Controller LONGITUDINAL/PF Yaw Channel L1 Augmentation/State predictor ==
  u2 : Inport
  sighat_2 : Inport  Port=2
  Integrator2 : Integrator
  ON : Constant  Value=m
  Product : Product  RndMeth=Zero
  Sum1 : Sum  Inputs=|++
  Sum2 : Sum  Inputs=|+-
  u_psi_hat : Outport
  wires:
  ON/1 -> Product/1
  Product/1 -> Integrator2/1
  Sum2/1 -> Product/2
  Integrator2/1 -> Sum2/2, u_psi_hat/1
  u2/1 -> Sum1/1
  Sum1/1 -> Sum2/1
  sighat_2/1 -> Sum1/2

== system AttitudeComplementary2/Plant Model/Plant/6-DOF EOM ==
  "[F,M]" : Inport
  Vb Corr : Inport  Orientation=left  Port=2
  Angular Rates : Integrator  InitialCondition=PQR_0'
  Demux1 : Demux  Outputs=[3 3]
  Euler Angles : Integrator  InitialCondition=Euler_0'
  Get Euler Dot : Subsystem
      mask Display:
      | port_label('input', 1, 'p, q, r')
      | port_label('input', 2, 'Euler')
      | port_label('output', 1, 'Euler_dot')
  Mux : Mux  Orientation=left  Inputs=[3;3]
  NED2NEU : Gain  Gain=[1 0 0;0 1 0;0 0 -1]  Multiplication=Matrix(K*u)  SaturateOnIntegerOverflow=on
  Position : Integrator  InitialCondition=Pos_0'
  RB2L * Vb : Product  Multiplication=Matrix(*)  SaturateOnIntegerOverflow=on  InputSameDT=on
  RB2LTP : Subsystem
  Velocities Body : Integrator  InitialCondition=Vb_0'
  "[V1,2,3,W1,2,3]" : Subsystem
  X,Y,Z (LTP) : Outport
  "Vx, Vy, Vz" : Outport  Port=2
  Euler : Outport  Port=3
  "p, q, r" : Outport  Orientation=left  Port=4
  Euler_dot : Outport  Port=5
  Vb : Outport  Port=6
  Ab : Outport  Port=7
  Ab meas : Outport  Port=8
  wires:
  "[V1,2,3,W1,2,3]"/1("Acc_meas ") -> Ab meas/1
  Euler Angles/1 -> "[V1,2,3,W1,2,3]"/2(Euler), Get Euler Dot/2(Euler), Euler/1, RB2LTP/1(Euler)
  Demux1/1 -> Ab/1, Velocities Body/1
  "[V1,2,3,W1,2,3]"/2(V*dot) -> Demux1/1
  Demux1/2 -> Angular Rates/1
  "[F,M]"/1 -> "[V1,2,3,W1,2,3]"/1("[F ; M]")
  RB2LTP/1(Rot) -> RB2L * Vb/1
  Velocities Body/1 -> Vb/1, RB2L * Vb/2
  Mux/1 -> "[V1,2,3,W1,2,3]"/3(V*)
  Position/1 -> X,Y,Z (LTP)/1
  Angular Rates/1 -> Get Euler Dot/1(p,q,r), Mux/2, "p, q, r"/1
  RB2L * Vb/1 -> NED2NEU/1, "Vx, Vy, Vz"/1  "NED"
  NED2NEU/1 -> Position/1
  Get Euler Dot/1(Euler_dot) -> Euler Angles/1, Euler_dot/1
  Vb Corr/1 -> Mux/1

== system AttitudeComplementary2/Plant Model/Plant/Engine Model ==
  dt : Inport
  Vmag : Inport  Port=2
  Constant4 : Constant  Value=0
  Get To1 : Subsystem
  Mux : Mux  Inputs=2
  Mux1 : Mux  Inputs=3
  Thrust Available (lbs) : Fcn  Expr=u(1) - 0.047*sqrt(u(1))*u(2)
  kg2N : Gain  Gain=ISA_g  SaturateOnIntegerOverflow=on
  lbs2kg : Gain  Gain=0.45359237  SaturateOnIntegerOverflow=on
  RPM : Outport
  Thrust : Outport  Port=2
  wires:
  Get To1/1(RPM) -> RPM/1
  dt/1 -> Get To1/1(dt)
  Get To1/2(To) -> Mux/1
  Mux/1 -> Thrust Available (lbs)/1
  Thrust Available (lbs)/1 -> lbs2kg/1
  Vmag/1 -> Mux/2
  Mux1/1 -> Thrust/1
  lbs2kg/1 -> kg2N/1
  Constant4/1 -> Mux1/2, Mux1/3
  kg2N/1 -> Mux1/1

== system AttitudeComplementary2/Plant Model/Plant/Forces and Moments ==
  Wind e : Inport
  Rho : Inport  Port=2
  "de, deg" : Inport  Port=3
  da,deg : Inport  Port=4
  "dr, deg" : Inport  Port=5
  "df, deg" : Inport  Port=6
  "Vx, Vy, Vz " : Inport  Port=7
  Euler : Inport  Port=8  PortDimensions=3
  p,q,r : Inport  Port=9
  Alpha/Beta : Subsystem
  Body Frame F & M : Subsystem
  Get Grav Force in Body : Subsystem
  Gravitational Force : Constant  Value=[0 0 mass*ISA_g]  VectorParams1D=off
  Mux : Mux  Inputs=2
  Mux1 : Mux  Inputs=2
  NED(u)2b : Subsystem
  Scope : Scope
      settings: SaveName=ScopeData5
  Selector : Selector  IndexOptions=Index vector (dialog)  Indices=3  OutputSizes=1  InputPortWidth=3
  Selector1 : Selector  Orientation=up  IndexOptions=Index vector (dialog)  Indices=3  OutputSizes=1  InputPortWidth=3
  Sum : Sum  Inputs=|++  SaturateOnIntegerOverflow=on
  Vair : Sum  Inputs=+-  SaturateOnIntegerOverflow=on  InputSameDT=on
  Airspeed : Outport
  Forces : Outport  Port=2
  Moments : Outport  Port=3
  Vb Corr : Outport  Port=4
  "aoa/betta, deg" : Outport  Port=5
  q : Outport  Port=6
  wires:
  Get Grav Force in Body/1(Grav Force (Body)) -> Sum/2
  Selector1/1 -> Mux1/2
  Mux1/1 -> Scope/1
  Selector/1 -> Mux1/1
  Mux/1 -> "aoa/betta, deg"/1
  Alpha/Beta/5(q) -> q/1
  "Vx, Vy, Vz "/1 -> Vair/1
  Vair/1 -> NED(u)2b/1(V w)
  Euler/1 -> NED(u)2b/2(Euler), Get Grav Force in Body/1(Euler)
  Rho/1 -> Alpha/Beta/2(Rho)
  NED(u)2b/1(Vb Corr) -> Alpha/Beta/1("Vx, Vy, Vz (Body)"), Vb Corr/1
  Body Frame F & M/2(M_b) -> Moments/1
  Gravitational Force/1 -> Get Grav Force in Body/2(Grav Force)
  Body Frame F & M/1(F_b) -> Selector/1, Sum/1
  Sum/1 -> Selector1/1, Forces/1
  Alpha/Beta/3(qS) -> Body Frame F & M/3(qs)
  Alpha/Beta/4(Speed) -> Body Frame F & M/4(Airspeed), Airspeed/1
  "df, deg"/1 -> Body Frame F & M/8("df, deg")
  p,q,r/1 -> Body Frame F & M/9(p,q,r)
  Alpha/Beta/2("beta, deg") -> Mux/2, Body Frame F & M/2("Beta, deg")
  "dr, deg"/1 -> Body Frame F & M/7("dr, deg")
  da,deg/1 -> Body Frame F & M/6("da, deg")
  Alpha/Beta/1("alpha, deg") -> Mux/1, Body Frame F & M/1("Alpha, deg")
  "de, deg"/1 -> Body Frame F & M/5("de, deg")
  Wind e/1 -> Vair/2

== system AttitudeComplementary2/Plant Model/Plant/Get GPS ==
  XYZ (NEU) : Inport
  Angle Conversion : aerolibconvert2/Angle Conversion  SystemSampleTime=-1  IU=deg  OU=rad
  Demux : Demux  Outputs=6
  Demux2 : Demux  Outputs=2
  Flat Earth to LLA : aerolibtransform2/Flat Earth to LLA  SystemSampleTime=-1  units=Metric (MKS)  ptype=Earth (WGS84)  F=1/298.257223563  R=6378137  LL0=[37.0004768371582, -122.061897277832]  psi=0
  MATLAB Fcn : MATLABFcn  MATLABFcn=u(1)*clock  OutputSignalType=real
  NEU2NED : Gain  Gain=[1 0 0;0 1 0;0 0 -1]  Multiplication=Matrix(K*u)  SaturateOnIntegerOverflow=on
  Rounding Function : Rounding
  Zero level trust : Constant  Value=0
  Zero level trust1 : Constant
  Zero level trust2 : Constant  Value=0
  GPS Month : Outport
  GPS Day : Outport  Port=2
  GPS Year : Outport  Port=3
  GPS Hr : Outport  Port=4
  GPS Min : Outport  Port=5
  GPS Sec : Outport  Port=6
  GPS Frac Sec : Outport  Port=7
  GPS Lat (rad) : Outport  Port=8
  GPS Long (rad) : Outport  Port=9
  GPS H (m) : Outport  Port=10
  wires:
  NEU2NED/1 -> Flat Earth to LLA/1
  Zero level trust/1 -> Flat Earth to LLA/2
  XYZ (NEU)/1 -> NEU2NED/1
  Flat Earth to LLA/1 -> Angle Conversion/1
  Flat Earth to LLA/2 -> GPS H (m)/1
  Zero level trust1/1 -> MATLAB Fcn/1
  MATLAB Fcn/1 -> Demux/1
  Demux/2 -> GPS Month/1
  Demux/3 -> GPS Day/1
  Demux/1 -> GPS Year/1
  Demux/4 -> GPS Hr/1
  Demux/5 -> GPS Min/1
  Demux/6 -> Rounding Function/1
  Rounding Function/1 -> GPS Sec/1
  Zero level trust2/1 -> GPS Frac Sec/1
  Angle Conversion/1 -> Demux2/1
  Demux2/1 -> GPS Lat (rad)/1
  Demux2/2 -> GPS Long (rad)/1

== system AttitudeComplementary2/Plant Model/Plant/ISA Atmosphere & Winds ==
  "X, Y, Z" : Inport
  Correct Wind : Constant  Value=[0;0;0]
  Get Z : Selector  IndexOptions=Index vector (dialog)  Indices=[3]  OutputSizes=[(-2)]  InputPortWidth=3
  ISA Atmosphere Model1 : aerolibatmos2/ISA Atmosphere Model  SystemSampleTime=-1  custom=off  g=9.80665  gamma=1.4  R=287.0531  L=0.0065  h_trop=11000  h_strat=20000  rho0=1.225  P0=101325  T0=288.15
  Terminator : Terminator
  Terminator1 : Terminator
  Rho : Outport
  Wind : Outport  Port=2
  AirPressure (Pa) : Outport  Port=3
  wires:
  "X, Y, Z"/1 -> Get Z/1
  Get Z/1 -> ISA Atmosphere Model1/1
  ISA Atmosphere Model1/4 -> Rho/1
  ISA Atmosphere Model1/1 -> Terminator/1
  ISA Atmosphere Model1/2 -> Terminator1/1
  ISA Atmosphere Model1/3 -> AirPressure (Pa)/1
  Correct Wind/1 -> Wind/1
